simulink model "Selecao_Otima_BFT2"  (R2025b)
settings: Solver=ode1  StartTime=0.0  StopTime=10.0  RelTol=1e-3
undefined symbols (not defined in the file or in its folder): Chapallaz_otimizado, Chapallaz_selecao, coef_eff, coef_head, Densidade1, Gravidade1, Ht1, Ht1_opt, Qt3_m3s, Qt3_opt_m3s, Rendimento_BFT1, Rendimento_BFT1_opt, Rendimento_Gerador1
libraries: simulink x1
settings Model: LastModifiedBy=guest

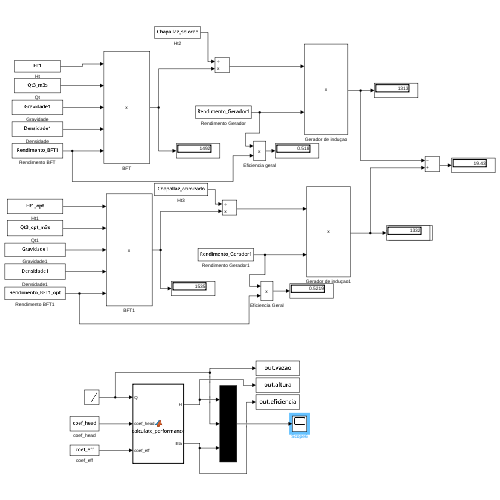
[thumbnail: Simulink's stored preview of the top-level diagram]
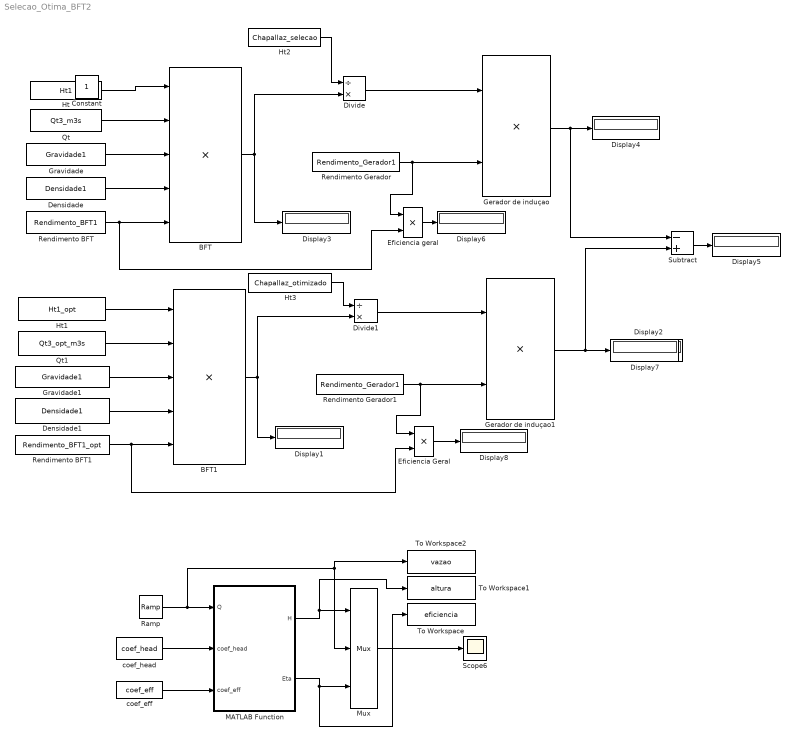
== system Selecao_Otima_BFT2 ==
  BFT : Product  Inputs=5
  BFT1 : Product  Inputs=5
  Densidade : Constant  Value=Densidade1
  Densidade1 : Constant  Value=Densidade1
  Display{1..8} (8 alike) : Display
  Divide : Product  Inputs=/*
  Divide1 : Product  Inputs=/*
  Eficiencia Geral : Product
  Eficiencia geral : Product
  Gerador de induçao : Product
  Gerador de induçao1 : Product
  Gravidade : Constant  Value=Gravidade1
  Gravidade1 : Constant  Value=Gravidade1
  Ht : Constant  Value=Ht1
  Ht1 : Constant  Value=Ht1_opt
  Ht2 : Constant  Value=Chapallaz_selecao
  Ht3 : Constant  Value=Chapallaz_otimizado
  MATLAB Function : MATLAB Function  TreatAsAtomicUnit=on
  Mux : Mux  Inputs=3
  Qt : Constant  Value=Qt3_m3s
  Qt1 : Constant  Value=Qt3_opt_m3s
  Ramp : simulink/Sources/Ramp  slope=5  start=0  InitialOutput=11.5
  Rendimento BFT : Constant  Value=Rendimento_BFT1
  Rendimento BFT1 : Constant  Value=Rendimento_BFT1_opt
  Rendimento Gerador : Constant  Value=Rendimento_Gerador1
  Rendimento Gerador1 : Constant  Value=Rendimento_Gerador1
  Scope6 : Scope
      settings: ActiveDisplayYMinimum=35.5499273912866  ActiveDisplayYMaximum=77.555810133946508
  Subtract : Sum  Inputs=-+
  To Workspace : ToWorkspace  VariableName=eficiencia  SaveFormat=Timeseries  SampleTime=-1
  To Workspace1 : ToWorkspace  VariableName=altura  SaveFormat=Timeseries  SampleTime=-1
  To Workspace2 : ToWorkspace  VariableName=vazao  SaveFormat=Timeseries  SampleTime=-1
  coef_eff : Constant  Value=coef_eff
  coef_head : Constant  Value=coef_head
  Constant : Constant  IOType=siggen
  wires:
  Rendimento Gerador/1 -> Eficiencia geral/1, Gerador de induçao/2
  BFT/1 -> Divide/2, Display3/1
  Gerador de induçao/1 -> Subtract/1, Display4/1
  Rendimento BFT/1 -> Eficiencia geral/2, BFT/5
  Densidade/1 -> BFT/4
  Gravidade/1 -> BFT/3
  Qt/1 -> BFT/2
  Ht/1 -> BFT/1
  Mux/1 -> Scope6/1
  Ramp/1 -> To Workspace2/1, Mux/2, MATLAB Function/1(Q)
  coef_head/1 -> MATLAB Function/2(coef_head)
  coef_eff/1 -> MATLAB Function/3(coef_eff)
  MATLAB Function/1(H) -> To Workspace1/1, Mux/1
  MATLAB Function/2(Eta) -> To Workspace/1, Mux/3
  Ht1/1 -> BFT1/1
  Gerador de induçao1/1 -> Display7/1, Subtract/2
  Rendimento BFT1/1 -> Eficiencia Geral/2, BFT1/5
  Rendimento Gerador1/1 -> Eficiencia Geral/1, Gerador de induçao1/2
  Qt1/1 -> BFT1/2
  Gravidade1/1 -> BFT1/3
  BFT1/1 -> Divide1/2, Display1/1
  Densidade1/1 -> BFT1/4
  Subtract/1 -> Display5/1
  Eficiencia geral/1 -> Display6/1
  Eficiencia Geral/1 -> Display8/1
  Divide1/1 -> Gerador de induçao1/1
  Divide/1 -> Gerador de induçao/1
  Ht2/1 -> Divide/1
  Ht3/1 -> Divide1/1

== matlab function Selecao_Otima_BFT2/MATLAB Function ==
  data: H output; Eta output; Q input; coef_head input; coef_eff input
function [H, Eta] = calculate_performance(Q, coef_head, coef_eff)
%Define a constante K

K_P = 0.0027252777777;

% 1 Altura
H = polyval(coef_head, Q);

%Eficiencia
Eta_perc = polyval (coef_eff, Q);
Eta_dec = Eta_perc / 100.0;

%3. Potencia no eixo
P_eixo = K_P * Q .* H .* Eta_dec;

Eta = Eta_perc; 
%Retorna eficiencia em porcentagem
end
